simulink library "magnetorquer_assembly_firstorder_lib"  (R2016b)
settings: Solver=VariableStepAuto  StartTime=0.0  StopTime=10.0  RelTol=1e-3
undefined symbols (not defined in the file or in its folder): sim_params
libraries: magnetorquer_lib x3
settings Model: Creator=Taylor  LastModifiedBy=taylorreynolds

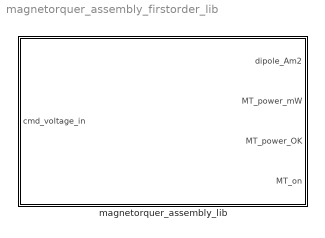
== system magnetorquer_assembly_firstorder_lib ==
  magnetorquer_assembly_lib : Subsystem

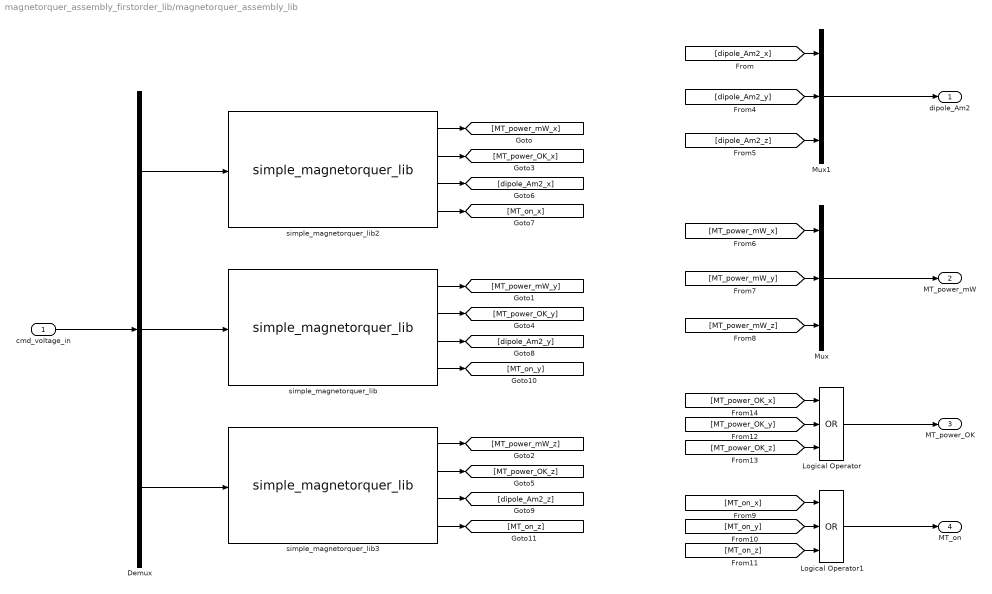
== system magnetorquer_assembly_firstorder_lib/magnetorquer_assembly_lib ==
  cmd_voltage_in : Inport
  Demux : Demux  Outputs=3
  Logical Operator : Logic  Operator=OR  Inputs=3  AllPortsSameDT=off  OutDataTypeStr=boolean
  Logical Operator1 : Logic  Operator=OR  Inputs=3  AllPortsSameDT=off  OutDataTypeStr=boolean
  Mux : Mux  Inputs=3
  Mux1 : Mux  Inputs=3
  simple_magnetorquer_lib : magnetorquer_lib/simple_magnetorquer_lib  A=sim_params.actuators.magnetorquer.area_y  N=sim_params.actuators.magnetorquer.num_turns_y  mu=sim_params.actuators.magnetorquer.mu_y  Linv=1/sim_params.actuators.magnetorquer.inductance_y  R=sim_params.actuators.magnetorquer.resistance_y  UpperLimit=sim_params.actuators.magnetorquer.max_dipole_y  LowerLimit=-sim_params.actuators.magnetorquer.max_dipole_y
  simple_magnetorquer_lib2 : magnetorquer_lib/simple_magnetorquer_lib  A=sim_params.actuators.magnetorquer.area_x  N=sim_params.actuators.magnetorquer.num_turns_x  mu=sim_params.actuators.magnetorquer.mu_x  Linv=1/sim_params.actuators.magnetorquer.inductance_x  R=sim_params.actuators.magnetorquer.resistance_x  UpperLimit=sim_params.actuators.magnetorquer.max_dipole_x  LowerLimit=-sim_params.actuators.magnetorquer.max_dipole_x
  simple_magnetorquer_lib3 : magnetorquer_lib/simple_magnetorquer_lib  A=sim_params.actuators.magnetorquer.area_z  N=sim_params.actuators.magnetorquer.num_turns_z  mu=sim_params.actuators.magnetorquer.mu_z  Linv=1/sim_params.actuators.magnetorquer.inductance_z  R=sim_params.actuators.magnetorquer.resistance_z  UpperLimit=sim_params.actuators.magnetorquer.max_dipole_z  LowerLimit=-sim_params.actuators.magnetorquer.max_dipole_z
  dipole_Am2 : Outport
  MT_power_mW : Outport  Port=2
  MT_power_OK : Outport  Port=3
  MT_on : Outport  Port=4
  wires:
  simple_magnetorquer_lib3/1 -> [MT_power_mW_z]
  simple_magnetorquer_lib2/1 -> [MT_power_mW_x]
  [dipole_Am2_y] -> Mux1/2
  [MT_power_mW_x] -> Mux/1
  [MT_on_x] -> Logical Operator1/1
  simple_magnetorquer_lib2/2 -> [MT_power_OK_x]
  simple_magnetorquer_lib2/3 -> [dipole_Am2_x]
  simple_magnetorquer_lib/2 -> [MT_power_OK_y]
  Demux/2 -> simple_magnetorquer_lib/1
  Demux/1 -> simple_magnetorquer_lib2/1
  simple_magnetorquer_lib/4 -> [MT_on_y]
  [dipole_Am2_x] -> Mux1/1
  simple_magnetorquer_lib/3 -> [dipole_Am2_y]
  simple_magnetorquer_lib3/2 -> [MT_power_OK_z]
  simple_magnetorquer_lib3/3 -> [dipole_Am2_z]
  simple_magnetorquer_lib3/4 -> [MT_on_z]
  Mux1/1 -> dipole_Am2/1
  [dipole_Am2_z] -> Mux1/3
  [MT_power_OK_z] -> Logical Operator/3
  [MT_on_y] -> Logical Operator1/2
  [MT_power_OK_y] -> Logical Operator/2
  [MT_power_mW_y] -> Mux/2
  [MT_on_z] -> Logical Operator1/3
  [MT_power_mW_z] -> Mux/3
  [MT_power_OK_x] -> Logical Operator/1
  Logical Operator/1 -> MT_power_OK/1
  Mux/1 -> MT_power_mW/1
  Logical Operator1/1 -> MT_on/1
  cmd_voltage_in/1 -> Demux/1
  simple_magnetorquer_lib2/4 -> [MT_on_x]
  simple_magnetorquer_lib/1 -> [MT_power_mW_y]
  Demux/3 -> simple_magnetorquer_lib3/1
